simulink model "sla_FFT"  (R2015b)
settings: Solver=FixedStepDiscrete  SolverMode=SingleTasking  StartTime=0.0  StopTime=simTime  RelTol=1e-3
PreLoadFcn:
  | paramFFTShift
values from neighbouring files (symbols this model uses):
  addrOffst = fi(N/2, 0, ceil(log2(N/2+1)), 0)    [paramFFTShift.m]
  addrWidth = uint16(log2(N))    [paramFFTShift.m]
  countMax = fi(4095, 0, ceil(log2(4095+1)), 0)    [paramFFTShift.m]
  countMax2 = fi(6144, 0, ceil(log2(6144+1)), 0)    [paramFFTShift.m]
  fftLatency = 559    [paramFFTShift.m]
  inputSignalFreq = [320 810 1290]    [paramFFTShift.m]
  N = 1024    [paramFFTShift.m]
  sr = 10e3    (= 10000)    [paramFFTShift.m]
undefined symbols (not defined in the file or in its folder): Radix
libraries: dspsrcs4 x2, dspxfrm3 x2, hdlsllib x2
settings Model: DataTypeOverride=Off  Creator=Aiko  LastModifiedBy=amatsumo
settings SolverCC: AutoInsertRateTranBlk=on
settings DataIOCC: SaveFormat=Array  SaveOutput=off  SaveTime=off
settings OptimizationCC: BlockReduction=off  ConditionallyExecuteInputs=off  DefaultParameterBehavior=Inlined
settings DebuggingCC: AlgebraicLoopMsg=error  UnderspecifiedInitializationDetection=Classic  MergeDetectMultiDrivingBlocksExec=none  SolverPrmCheckMsg=warning  SingleTaskRateTransMsg=error
settings HardwareCC: ProdBitPerPointer=32  ProdLargestAtomicFloat=None  ProdIntDivRoundTo=Undefined  ProdEndianess=Unspecified  ProdWordSize=32  ProdHWDeviceType=ASIC/FPGA->ASIC/FPGA  ProdEqTarget=off
settings GRTTargetCC: GeneratePreprocessorConditionals=Disable all
settings ConfigComp: CovModelRefEnable=Off  CovSFcnEnable=off

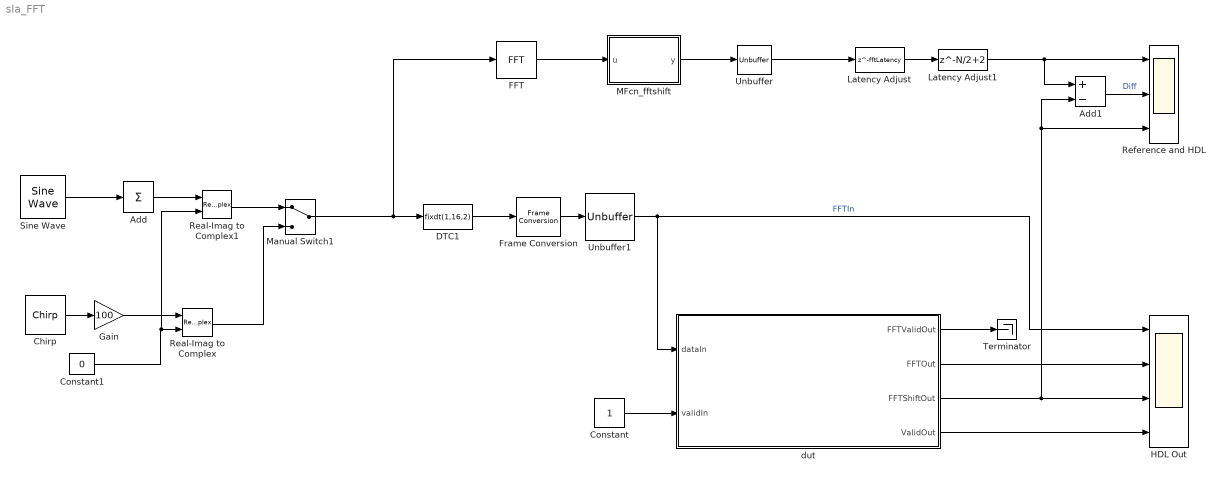
== system sla_FFT ==
  Add : Sum  Inputs=+  CollapseMode=Specified dimension  CollapseDim=2
  Add1 : Sum  Inputs=+-
  Chirp : dspsrcs4/Chirp  sweep=Linear  mode=Unidirectional  f0=500  f1=3200  t1=N/sr  Tsweep=N/sr  phase=0  Ts=1/sr  spf=N  datatype=Double  OutputFrames=on
  Constant : Constant  OutDataTypeStr=boolean  SampleTime=1/sr
  Constant1 : Constant  Value=0  OutDataTypeStr=Inherit: Inherit via back propagation  SampleTime=-1
  DTC1 : DataTypeConversion  OutDataTypeStr=fixdt(1,16,2)  RndMeth=Nearest  SaturateOnIntegerOverflow=on
  FFT : dspxfrm3/FFT  FFTImplementation=Radix-2  CompMethod=Table lookup  TableOpt=NEW  TableOptActive=Speed  BitRevOrder=off  Normalize=off  InheritFFTLength=off  FFTLength=N  WrapInput=on  roundingMode=Floor  overflowMode=off  firstCoeffDataTypeStr=Inherit: Same word length as input  firstCoeffLastDataTypeStr=Inherit: Same word length as input  outputMin=[]  outputMax=[]
  Frame Conversion : FrameConversion  InheritSamplingMode=off
  Gain : Gain  Gain=100
  HDL Out : Scope  NumInputPorts=4
  Latency Adjust : Delay  DelayLength=fftLatency
  Latency Adjust1 : Delay  DelayLength=N/2+2
  MFcn_fftshift : MATLAB Function  TreatAsAtomicUnit=on
  Manual Switch1 : ManualSwitch
  Real-Imag to Complex : RealImagToComplex
  Real-Imag to Complex1 : RealImagToComplex
  Reference and HDL : Scope  NumInputPorts=3
  Sine Wave : dspsrcs4/Sine Wave  Amplitude=5  Frequency=inputSignalFreq  Phase=0  SampleMode=Discrete  OutComplex=Real  CompMethod=Trigonometric fcn  TableSize=Speed  SampleTime=1/sr  SamplesPerFrame=N  ResetState=Restart at time zero  OutputFrames=on  dataType=double  wordLen=16  udDataType=sfix(16)  fracBitsMode=Best precision  numFracBits=15  OutDataTypeStr=double  LastOutDataTypeStr=double
  Terminator : Terminator
  Unbuffer : Unbuffer  SampleBasedProcessing=Same as frame based
  Unbuffer1 : Unbuffer  SampleBasedProcessing=Same as frame based
  dut : Subsystem
  wires:
  Manual Switch1/1 -> FFT/1, DTC1/1
  Unbuffer1/1 -> dut/1(dataIn), HDL Out/1  "FFTIn"
  Add1/1 -> Reference and HDL/2  "Diff"
  Unbuffer/1 -> Latency Adjust/1
  Frame Conversion/1 -> Unbuffer1/1
  Sine Wave/1 -> Add/1
  DTC1/1 -> Frame Conversion/1
  FFT/1 -> MFcn_fftshift/1(u)
  Chirp/1 -> Gain/1
  Latency Adjust/1 -> Latency Adjust1/1
  Gain/1 -> Real-Imag to Complex/1
  Latency Adjust1/1 -> Add1/1, Reference and HDL/1
  MFcn_fftshift/1(y) -> Unbuffer/1
  Real-Imag to Complex/1 -> Manual Switch1/2
  Add/1 -> Real-Imag to Complex1/1
  Constant1/1 -> Real-Imag to Complex1/2, Real-Imag to Complex/2
  Real-Imag to Complex1/1 -> Manual Switch1/1
  dut/3(FFTShiftOut) -> HDL Out/3, Add1/2, Reference and HDL/3
  dut/2(FFTOut) -> HDL Out/2
  Constant/1 -> dut/2(validIn)
  dut/4(ValidOut) -> HDL Out/4
  dut/1(FFTValidOut) -> Terminator/1

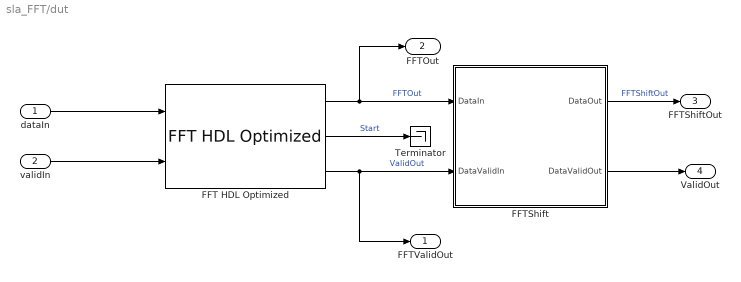
== system sla_FFT/dut ==
  dataIn : Inport
  validIn : Inport  Port=2
  FFT HDL Optimized : dspxfrm3/FFT HDL Optimized  BitReversedOutput=off  Normalize=off  FFTLengthSource=Property  FFTLength=N  RoundingMethod=Floor  OverflowAction=Saturate  ValidInputPort=on  ResetInputPort=off  StartOutputPort=on  EndOutputPort=off  SimulateUsing=Code generation
  FFTShift : Subsystem
  Terminator : Terminator
  FFTValidOut : Outport
  FFTOut : Outport  Port=2
  FFTShiftOut : Outport  Port=3
  ValidOut : Outport  Port=4
  wires:
  FFT HDL Optimized/1 -> FFTShift/1(DataIn), FFTOut/1  "FFTOut"
  FFTShift/1(DataOut) -> FFTShiftOut/1  "FFTShiftOut"
  FFT HDL Optimized/3 -> FFTValidOut/1, FFTShift/2(DataValidIn)  "ValidOut"
  FFT HDL Optimized/2 -> Terminator/1  "Start"
  validIn/1 -> FFT HDL Optimized/2
  FFTShift/2(DataValidOut) -> ValidOut/1
  dataIn/1 -> FFT HDL Optimized/1

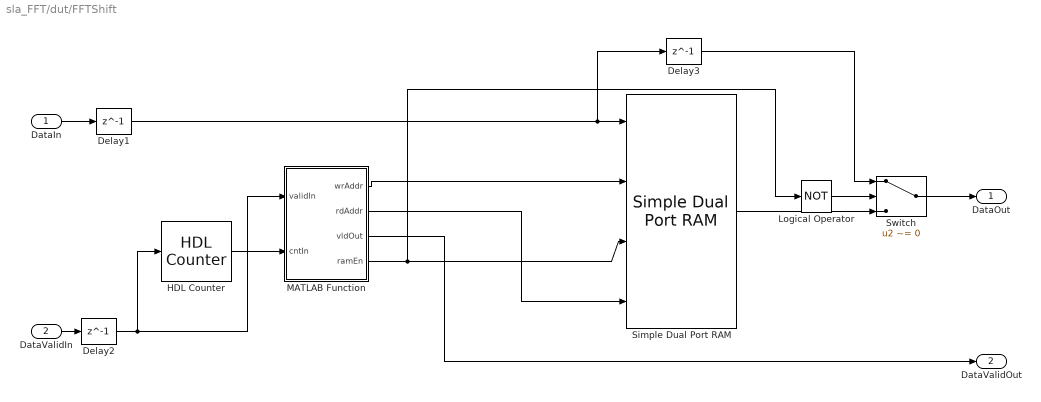
== system sla_FFT/dut/FFTShift ==
  DataIn : Inport
  DataValidIn : Inport  Port=2
  Delay1 : Delay  DelayLength=1
  Delay2 : Delay  DelayLength=1
  Delay3 : Delay  DelayLength=1
  HDL Counter : hdlsllib/HDL Operations/HDL Counter  CountType=Count limited  CountInit=0  CountStep=1  CountMax=N-1  CountFromType=Initial value  CountFrom=0  CountResetPort=off  CountLoadPort=off  CountEnbPort=on  CountDirPort=off  CountDataType=Unsigned  CountWordLen=log2(N)  CountFracLen=0  CountSampTime=1
  Logical Operator : Logic  Operator=NOT  AllPortsSameDT=off  OutDataTypeStr=boolean
  MATLAB Function : MATLAB Function  TreatAsAtomicUnit=on
  Simple Dual Port RAM : hdlsllib/HDL Operations/Simple Dual Port RAM  ram_size=log2(N)
  Switch : Switch  Criteria=u2 ~= 0
  DataOut : Outport
  DataValidOut : Outport  Port=2
  wires:
  MATLAB Function/3(vldOut) -> DataValidOut/1
  MATLAB Function/2(rdAddr) -> Simple Dual Port RAM/4
  MATLAB Function/1(wrAddr) -> Simple Dual Port RAM/2
  DataValidIn/1 -> Delay2/1
  DataIn/1 -> Delay1/1
  Delay2/1 -> HDL Counter/1, MATLAB Function/1(validIn)
  Switch/1 -> DataOut/1
  Simple Dual Port RAM/1 -> Switch/3
  Delay1/1 -> Delay3/1, Simple Dual Port RAM/1
  MATLAB Function/4(ramEn) -> Logical Operator/1, Simple Dual Port RAM/3
  HDL Counter/1 -> MATLAB Function/2(cntIn)
  Logical Operator/1 -> Switch/2
  Delay3/1 -> Switch/1

== matlab function sla_FFT/dut/FFTShift/MATLAB Function ==
  settings: fimath=hdlfimath
  data: validIn input; cntIn input; wrAddr output; rdAddr output; vldOut output; addrWidth parameter; countMax parameter; countMax2 parameter; addrOffst parameter; ramEn output
function [wrAddr, rdAddr, vldOut, ramEn] = fcn(validIn, cntIn, addrWidth, countMax, countMax2, addrOffst)
%#codegen

persistent wrAddrCnt rdAddrCnt vldOutReg wrEnReg

if isempty(wrAddrCnt)
    wrAddrCnt      = fi(0, 0, addrWidth, 0);
    rdAddrCnt      = fi(addrOffst, 0, addrWidth, 0);
    wrEnReg     = true;
    vldOutReg   = false;
end

vldOut = vldOutReg;
wrAddr = wrAddrCnt;
rdAddr = rdAddrCnt;


if validIn
    vldOutReg = true;
    if (cntIn < addrOffst)
        rdAddrCnt = fi(rdAddrCnt + 1, 0, addrWidth, 0);
        wrAddrCnt = fi(wrAddrCnt + 1, 0, addrWidth, 0);
        wrEnReg = true;
    elseif (cntIn > countMax)&&(cntIn < countMax2)
        rdAddrCnt = fi(rdAddrCnt + 1, 0, addrWidth, 0);
        wrAddrCnt = fi(wrAddrCnt + 1, 0, addrWidth, 0);
        wrEnReg = true;
    else
        wrEnReg = false;
    end
    
    if rdAddrCnt > countMax
        rdAddrCnt      = fi(0, 0, addrWidth, 0);
    end
    if wrAddrCnt > countMax
        wrAddrCnt      = fi(0, 0, addrWidth, 0);
    end
    
else
    vldOutReg = false;
end
ramEn = wrEnReg;

== matlab function sla_FFT/MFcn_fftshift ==
  data: u input; y output
function y = fcn(u)
%#codegen

y = fftshift(u) ;

% y = u;
